simulink model "filter_current"  (R2023a)
settings: Solver=FixedStepDiscrete  StartTime=0.0  StopTime=10.0  FixedStep=FilterCurrent_Ts  RelTol=1e-3  EnableMultiTasking=on
model workspace (MAT data in the model file):
  FilterCurrent_Ts = Simulink.Parameter
  FilterCurrent_Ts.Value = 0.001
  FilterCurrent_Ts.DataType = 'auto'
  FilterCurrent_Ts.DocUnits = 's'
  FilterCurrent_Ts.Complexity = 'real'
  FilterCurrent_Ts.Dimensions = [1 1]
libraries: dspstat3 x1
settings Model: DataDictionary=EmbeddedBoardDD.sldd  Creator=ascalzo  LastModifiedBy=upattacini
settings SolverCC: AllowMultiTaskInputOutput=on  AutoInsertRateTranBlk=on  InsertRTBMode=Never (minimum delay)
settings DataIOCC: SaveOutput=off  SignalLogging=off  DSMLogging=off  SaveTime=off  ReturnWorkspaceOutputs=off
settings OptimizationCC: DefaultParameterBehavior=Inlined  DefaultUnderspecifiedDataType=single  StrengthReduction=on  PassReuseOutputArgsAs=Individual arguments  OptimizeBlockOrder=speed  OptimizationPriority=Speed  OptimizationCustomize=off  MultiThreadedLoops=on  EfficientTunableParamExpr=on
settings DebuggingCC: ParameterPrecisionLossMsg=none  UnconnectedInputMsg=warning  UnconnectedOutputMsg=warning  UnconnectedLineMsg=warning
settings HardwareCC: ProdBitPerPointer=32  ProdBitPerSizeT=32  ProdBitPerPtrDiffT=32  ProdLargestAtomicInteger=Long  ProdLargestAtomicFloat=Double  ProdWordSize=32  ProdHWDeviceType=ARM Compatible->ARM Cortex-M
settings ModelReferenceCC: UpdateModelReferenceTargets=Force  EnableRefExpFcnMdlSchedulingChecks=on
settings SFSimCC: MATLABDynamicMemAlloc=off
settings RTWCC: Description=Embedded Coder  SystemTargetFile=ert.tlc  GenCodeOnly=on  PackageGeneratedCodeAndArtifacts=on  PackageName=filter_current  TemplateMakefile=ert_default_tmf  TargetLang=C++  DLArmComputeVersion=19.05
settings CodeAppCC: ForceParamTrailComments=on  IgnoreCustomStorageClasses=off  MaxIdLength=60  OperatorAnnotations=on  SimulinkDataObjDesc=on  SFDataObjDesc=on  InsertBlockDesc=on
settings ERTTargetCC: TargetLangStandard=C++03 (ISO)  CodeReplacementLibrary=ARM Cortex-M,iCubTech  GenerateSampleERTMain=on  CodeInterfacePackaging=Reusable function  InlinedParameterPlacement=NonHierarchical  RootIOFormat=Structure reference  ERTCustomFileTemplate=example_file_process.tlc

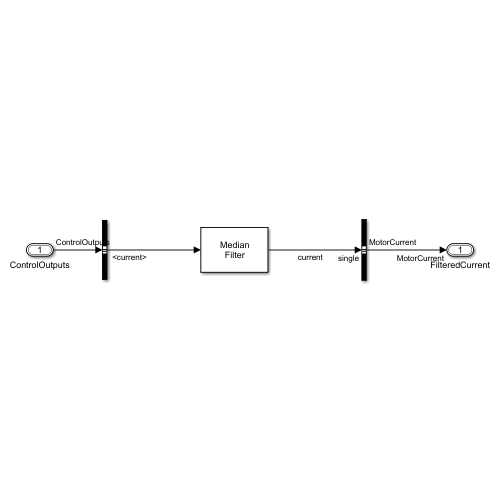
[thumbnail: Simulink's stored preview of the top-level diagram]
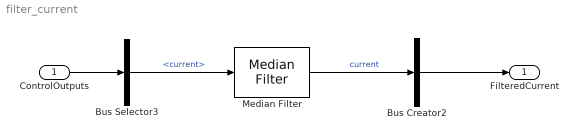
== system filter_current ==
  ControlOutputs : Inport  OutDataTypeStr=Bus: ControlOutputs  BusOutputAsStruct=on
  Bus Creator2 : BusCreator  Inputs=1  OutDataTypeStr=Bus: MotorCurrent  NonVirtualBus=on
      settings: InheritFromInputs=off
  Bus Selector3 : BusSelector  OutputSignals=Iq_fbk.current
  Median Filter : dspstat3/Median Filter  WindowLength=32  SimulateUsing=Code generation
  FilteredCurrent : Outport  OutDataTypeStr=Bus: MotorCurrent  BusOutputAsStruct=on
  wires:
  ControlOutputs/1 -> Bus Selector3/1
  Bus Creator2/1 -> FilteredCurrent/1
  Bus Selector3/1 -> Median Filter/1  "<current>"
  Median Filter/1 -> Bus Creator2/1  "current"
